simulink model "uORB_MODBUS_TCP"  (R2024a)
settings: Solver=FixedStepAuto  StartTime=0.0  StopTime=10.0  RelTol=1e-3  EnableMultiTasking=on
libraries: px4uORBlib x3
settings Model: ExtModeTrigDuration=10  Creator=root  LastModifiedBy=root
settings SolverCC: PositivePriorityOrder=on
settings OptimizationCC: OptimizeBlockIOStorage=off  BufferReuse=off  ReuseModelBlockBuffer=off  GlobalBufferReuse=off  ExpressionFolding=off  EnableMemcpy=off  PassReuseOutputArgsAs=Individual arguments  LocalBlockOutputs=off  ZeroExternalMemoryAtStartup=off  ZeroInternalMemoryAtStartup=off  MaxStackSize=64  OptimizeDataStoreBuffers=off  BusAssignmentInplaceUpdate=off  OptimizationLevel=level0  OptimizationCustomize=off  EfficientTunableParamExpr=on
settings DebuggingCC: ParameterTunabilityLossMsg=error
settings HardwareCC: ProdBitPerPointer=32  ProdBitPerSizeT=32  ProdBitPerPtrDiffT=32  ProdLargestAtomicInteger=Long  ProdLargestAtomicFloat=Double  ProdWordSize=32  ProdLongLongMode=on  ProdHWDeviceType=ARM Compatible->ARM Cortex
settings SFSimCC: SimUserSources=modbus_tcp_client.cpp  SimUserIncludeDirs=/home/judson/GSE-Miscellaneous/Pixhawk_and_GSE/MATLAB/uORB_MODBUS_TCP  MATLABDynamicMemAlloc=off  CustomCodeGlobalsAsFunctionIO=on  SimTargetLang=C++
settings SFSimCC: SimCustomHeaderCode=|
  | #include <netinet/in.h>
  | #include <sys/types.h>
  | #include <sys/socket.h>
  | #include <arpa/inet.h>
  | #include <errno.h>
  | #include <stdio.h>
  | #include <string.h>
  | #include <unistd.h>
  | #include "modbus_tcp_client.h"
settings RTWCC: Description=Embedded Coder  SystemTargetFile=ert.tlc  HardwareBoard=PX4 Pixhawk 6x  TLCOptions="-aInlineSetEventsForThisBaseRateFcn=TLC_FALSE -aSuppressMultiTaskScheduler=TLC_FALSE  -aRateBasedStepFcn=0"  TemplateMakefile=ert_default_tmf  RTWUseSimCustomCode=on  CustomInclude=/home/judson/GSE-Miscellaneous/Pixhawk_and_GSE/MATLAB/uORB_MODBUS_TCP  CustomSource=modbus_tcp_client.cpp  Toolchain=GNU Tools for PX4 Autopilots  BuildConfiguration=Debug  TargetLang=C++
settings RTWCC: CustomHeaderCode=|
  | #include <netinet/in.h>
  | #include <sys/types.h>
  | #include <sys/socket.h>
  | #include <arpa/inet.h>
  | #include <errno.h>
  | #include <stdio.h>
  | #include <string.h>
  | #include <unistd.h>
  | #include "modbus_tcp_client.h"
settings CodeAppCC: ForceParamTrailComments=on  IgnoreCustomStorageClasses=off  OperatorAnnotations=on  SimulinkDataObjDesc=on  SFDataObjDesc=on  MATLABFcnDesc=on  InsertBlockDesc=on  EnableCustomComments=on  ReqsInCode=on
settings ERTTargetCC: TargetLangStandard=C++11 (ISO)  SupportNonFinite=off  ExtModeTransport=3  ExtModeStaticAlloc=on  ExtModeStaticAllocSize=1024  ExtModeMexFile=ext_xcp  ExtModeIntrfLevel=Level2 - Open  PreserveIfCondition=on

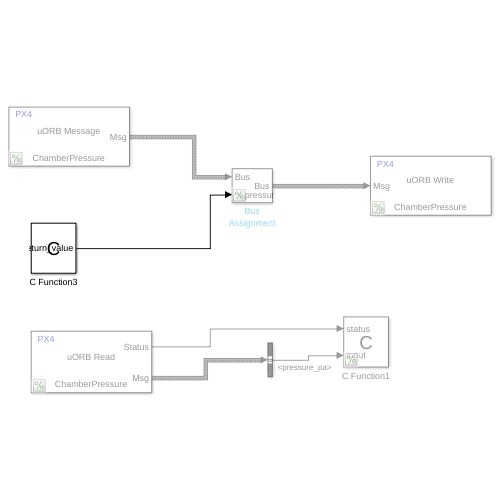
[thumbnail: Simulink's stored preview of the top-level diagram]
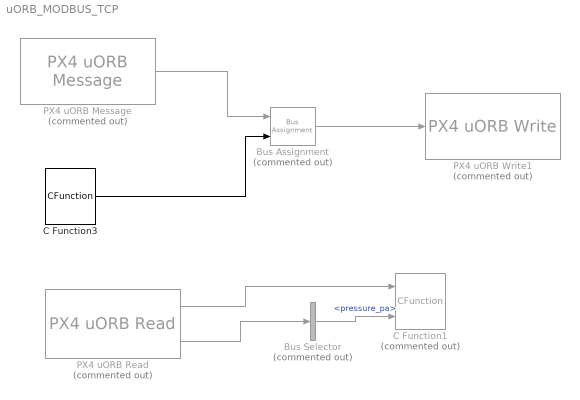
== system uORB_MODBUS_TCP ==
  Bus Assignment : BusAssignment  Commented=on  AssignedSignals=pressure_pa
  Bus Selector : BusSelector  Commented=on  OutputSignals=pressure_pa
  C Function1 : CFunction  Commented=on  OutputCode=|  CodegenOutputCode=|  SimCustomHeaderFile=""  CustomHeaderFile=""
      OutputCode=|
      | // printf("\n");
      | // printf("uORB Status: %d\n", status);
      | // printf("Register value: %.0f \n", input);
      CodegenOutputCode=|
      | // printf("\n");
      | // printf("uORB Status: %d\n", status);
      | // printf("Register value: %.0f \n", input);
  C Function3 : CFunction  OutputCode=|  CodegenOutputCode=|  SampleTime=5  SimCustomHeaderFile="#include \"modbus_tcp_client.h\""  CustomHeaderFile="#include \"modbus_tcp_client.h\""
      OutputCode=|
      | static ModbusTCPClient modbus("192.168.0.249", 5020, 10, 10, 10, 10);
      | 
      | if (!modbus.isConnected()) {
      |     modbus.setTimeout(1000);
      |     if (!modbus.connectServer()) {
      |         printf("Failed to connect to MODBUS server!\n");
      |         return;
      |     }
      | }
      | 
      | const int num_reads = 1000;
      | uint16_t last_value = 0;
      | uint16_t holdingRegisters[10] = {0};
      | float sum_differences = 0.0;
      | 
      | // Initial read to populate last_value
      | modbus.readMultipleHoldingRegisters(0, 10, holdingRegisters);
      | last_value = holdingRegisters[0];
      | 
      | // Loop 1000 times
      | for (int i = 0; i < num_reads; ++i) {
      |     modbus.readMultipleHoldingRegisters(0, 10, holdingRegisters);
      | 
      |     uint16_t current_value = holdingRegisters[0];
      | 
      |     // Handle 16-bit rollover
      |     uint16_t diff = (current_value >= last_value) 
      |                     ? (current_value - last_value) 
      |                     : (current_value + (65536 - last_value));
      | 
      |     sum_differences += (float)diff;
      | 
      |     last_value = current_value;
      | }
      | 
      | // Average the differences
      | float avg_diff = sum_differences / num_reads;
      | 
      | printf("Average time difference between reads (ms): %.2f\n", avg_diff);
      CodegenOutputCode=|
      | static ModbusTCPClient modbus("192.168.0.249", 5020, 10, 10, 10, 10);
      | 
      | if (!modbus.isConnected()) {
      |     modbus.setTimeout(1000);
      |     if (!modbus.connectServer()) {
      |         printf("Failed to connect to MODBUS server!\n");
      |         return;
      |     }
      | }
      | 
      | const int num_reads = 1000;
      | uint16_t last_value = 0;
      | uint16_t holdingRegisters[10] = {0};
      | float sum_differences = 0.0;
      | 
      | // Initial read to populate last_value
      | modbus.readMultipleHoldingRegisters(0, 10, holdingRegisters);
      | last_value = holdingRegisters[0];
      | 
      | // Loop 1000 times
      | for (int i = 0; i < num_reads; ++i) {
      |     modbus.readMultipleHoldingRegisters(0, 10, holdingRegisters);
      | 
      |     uint16_t current_value = holdingRegisters[0];
      | 
      |     // Handle 16-bit rollover
      |     uint16_t diff = (current_value >= last_value) 
      |                     ? (current_value - last_value) 
      |                     : (current_value + (65536 - last_value));
      | 
      |     sum_differences += (float)diff;
      | 
      |     last_value = current_value;
      | }
      | 
      | // Average the differences
      | float avg_diff = sum_differences / num_reads;
      | 
      | printf("Average time difference between reads (ms): %.2f\n", avg_diff);
  PX4 uORB Message : px4uORBlib/PX4 uORB Message  Commented=on  uORBTopic=ChamberPressure  SampleTime=-1  selectInstance=ChamberPressure
      settings: SourceProductName=PX4 uORB Read and Write Blocks
  PX4 uORB Read : px4uORBlib/PX4 uORB Read  Commented=on  uORBTopic=ChamberPressure  selectInstance=ChamberPressure  SampleTime=1  BlockingMode=off  BlockTimeout=1e-3
      settings: SourceProductName=PX4 uORB Read and Write Blocks
  PX4 uORB Write1 : px4uORBlib/PX4 uORB Write  Commented=on  uORBTopic=ChamberPressure  selectInstance=ChamberPressure  MessageQueueLen=1
      settings: SourceProductName=PX4 uORB Read and Write Blocks
  wires:
  PX4 uORB Message/1 -> Bus Assignment/1
  Bus Assignment/1 -> PX4 uORB Write1/1
  C Function3/1 -> Bus Assignment/2
  PX4 uORB Read/2 -> Bus Selector/1
  Bus Selector/1 -> C Function1/2  "<pressure_pa>"
  PX4 uORB Read/1 -> C Function1/1
